simulink model "APHLA40AFOCV2"  (R2018b)
settings: Solver=FixedStepAuto  StartTime=0.0  StopTime=10.0  RelTol=1e-3
settings Model: Creator=sweat  LastModifiedBy=39926

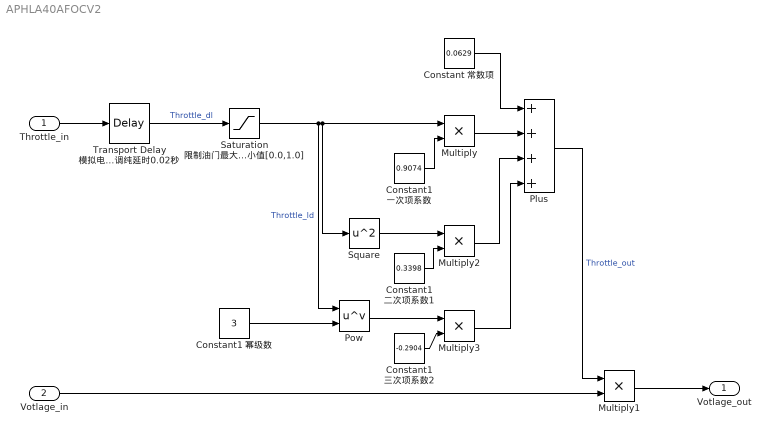
== system APHLA40AFOCV2 ==
  Throttle_in : Inport  PortDimensions=1
  Votlage_in : Inport  Port=2
  Constant 常数项 : Constant  Value=0.0629
  Constant1 一次项系数 : Constant  Value=0.9074
  Constant1 三次项系数2 : Constant  Value=-0.2904
  Constant1 二次项系数1 : Constant  Value=0.3398
  Constant1 幂级数 : Constant  Value=3
  Multiply{,1..3} (4 alike) : Product
  Plus : Sum  Inputs=++++
  Pow : Math  Operator=pow  RndMeth=Zero  SaturateOnIntegerOverflow=on
  Saturation 限制油门最大最小值[0.0,1.0] : Saturate  UpperLimit=1.0  LowerLimit=0.0
  Square : Math  Operator=square  SaturateOnIntegerOverflow=on
  Transport Delay 模拟电调纯延时0.02秒 : TransportDelay  DelayTime=0.02
  Votlage_out : Outport
  wires:
  Throttle_in/1 -> Transport Delay 模拟电调纯延时0.02秒/1
  Transport Delay 模拟电调纯延时0.02秒/1 -> Saturation 限制油门最大最小值[0.0,1.0]/1  "Throttle_dl"
  Saturation 限制油门最大最小值[0.0,1.0]/1 -> Pow/1, Square/1, Multiply/1  "Throttle_ld"
  Constant1 一次项系数/1 -> Multiply/2
  Multiply/1 -> Plus/2
  Constant 常数项/1 -> Plus/1
  Plus/1 -> Multiply1/1  "Throttle_out"
  Votlage_in/1 -> Multiply1/2
  Multiply1/1 -> Votlage_out/1
  Square/1 -> Multiply2/1
  Constant1 二次项系数1/1 -> Multiply2/2
  Constant1 幂级数/1 -> Pow/2
  Pow/1 -> Multiply3/1
  Constant1 三次项系数2/1 -> Multiply3/2
  Multiply2/1 -> Plus/3
  Multiply3/1 -> Plus/4
